simulink model "PTC_MBDS_DateTimeAssemble_Sample"  (R2013a)
settings: Solver=FixedStepDiscrete  StartTime=0.0  StopTime=Inf  FixedStep=0.01  RelTol=1e-3
libraries: PTC_MBDS_LIB x3, simulink_extras x2
settings Model: Creator=Jordan.Mosher  LastModifiedBy=Sundeep.Tuteja

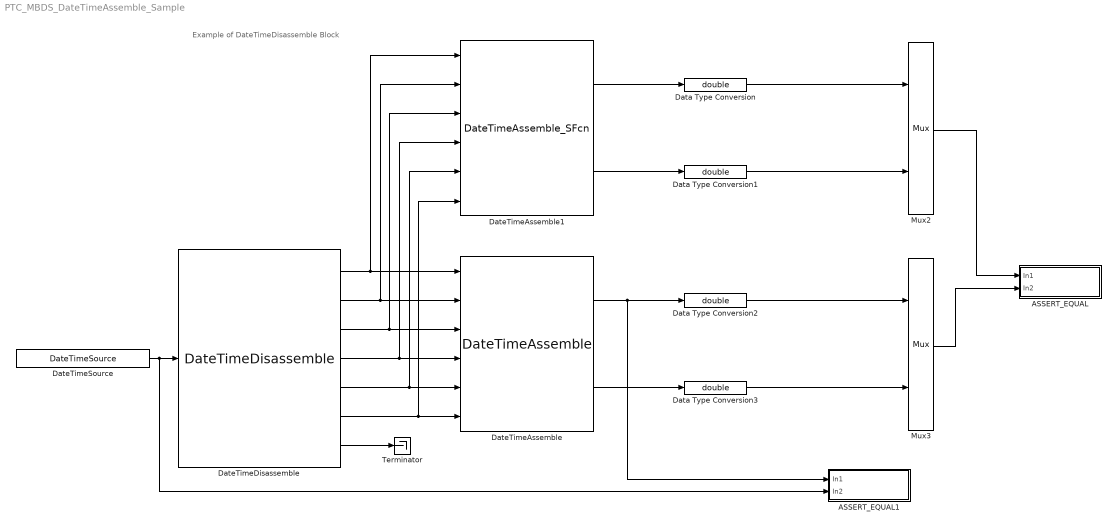
== system PTC_MBDS_DateTimeAssemble_Sample ==
  note: Example of DateTimeDisassemble Block
  ASSERT_EQUAL : Subsystem
  ASSERT_EQUAL1 : Subsystem
  Data Type Conversion{,1..3} (4 alike) : DataTypeConversion  OutDataTypeStr=double  SaturateOnIntegerOverflow=on
  DateTimeAssemble : PTC_MBDS_LIB/MBDS Standard Library/Extended Operations/Date & Time Operations/Date & Time Conversions/DateTimeAssemble  ENO_Enabled=on  PTC_MBDS_BlockVersion=5.40  PTC_BlockType=PTC_MBDS_DateTimeAssemble
  DateTimeAssemble1 : S-Function  InitFcn=|  FunctionName=DateTimeAssemble_SFcn  Parameters=boolean(ENO_Enabled)  EnableBusSupport=off  mask(DateTimeAssemble){MBDS_LibraryBlock=on, ENO_Enabled=on, MBDS_BlockVersion=05.40}
      | if(exist('MBDS_BlockCallback', 'file'))
      |    MBDS_BlockCallback('Update', gcb);  
      | end
      mask prompts: MBDS_LibraryBlock "MBDS Library Block"; ENO_Enabled "Show ENO port"; MBDS_BlockVersion "Block version:"
      mask help: Assembles a date_time signal from individual date and time components. The input values are restricted to their ranges (refer to the block help). If an input is out of range the ENO output is set to false.
      mask init:
      | MBDS_BlockCallback('Copy', gcb);     
      | maskdisplay = 'disp(sprintf(''Date Time\nAssemble''))';
      | maskdisplay = [maskdisplay 10 'port_label(''input'', 1, ''Year'')' 10];
      | maskdisplay = [maskdisplay 'port_label(''input'', 2, ''Month'')' 10];
      | maskdisplay = [maskdisplay 'port_label(''input'', 3, ''Day'')' 10];
      | maskdisplay = [maskdisplay 'port_label(''input'', 4, ''Hours'')' 10];
      | maskdisplay = [maskdisplay 'port_label(''input'', 5, ''Minutes'')' 10];
      | maskdisplay = [maskdisplay 'port_label(''input'', 6, ''Seconds'')' 10];
      | maskdisplay = [maskdisplay 'port_label(''output'', 1, ''DT'')' 10];
      | if(ENO_Enabled)
      |     maskdisplay = [maskdisplay 'port_label(''output'', 2, ''ENO'')' 10];
      | end
      | set_param(gcbh, 'maskdisplay', maskdisplay)
      mask Help: eval(['open([workdir(''RT_Dir:''),''\Host\Library\Blockset\Help\'',get_param(gcb,''MaskType''),''.html''])']);
      mask Display:
      | disp(sprintf('Date Time\nAssemble'))
      | port_label('input', 1, 'Year')
      | port_label('input', 2, 'Month')
      | port_label('input', 3, 'Day')
      | port_label('input', 4, 'Hours')
      | port_label('input', 5, 'Minutes')
      | port_label('input', 6, 'Seconds')
      | port_label('output', 1, 'DT')
      | port_label('output', 2, 'ENO')
  DateTimeDisassemble : PTC_MBDS_LIB/MBDS Standard Library/Extended Operations/Date & Time Operations/Date & Time Conversions/DateTimeDisassemble  ENO_Enabled=off  PTC_MBDS_BlockVersion=5.40  PTC_BlockType=PTC_MBDS_DateTimeDisassemble
  DateTimeSource : PTC_MBDS_LIB/MBDS Standard Library/Extended Operations/Date & Time Operations/DateTimeSource  InputValue=1986-12-01-12:55:13  PTC_MBDS_BlockVersion=5.40  PTC_BlockType=PTC_MBDS_DateTimeSource  Value=533825713
  Mux2 : Mux  Inputs=2
  Mux3 : Mux  Inputs=2
  Terminator : Terminator
      settings: InitFcn=|
      | try
      |    MBDS_BlockCallback('Update', gcb);
      | end
  wires:
  Mux3/1 -> ASSERT_EQUAL/2(In2)
  Mux2/1 -> ASSERT_EQUAL/1(In1)
  DateTimeDisassemble/7 -> Terminator/1
  DateTimeSource/1 -> ASSERT_EQUAL1/2(In2), DateTimeDisassemble/1
  DateTimeDisassemble/4 -> DateTimeAssemble1/4, DateTimeAssemble/4
  DateTimeDisassemble/5 -> DateTimeAssemble1/5, DateTimeAssemble/5
  DateTimeDisassemble/1 -> DateTimeAssemble1/1, DateTimeAssemble/1
  DateTimeDisassemble/2 -> DateTimeAssemble1/2, DateTimeAssemble/2
  DateTimeDisassemble/3 -> DateTimeAssemble1/3, DateTimeAssemble/3
  DateTimeDisassemble/6 -> DateTimeAssemble1/6, DateTimeAssemble/6
  DateTimeAssemble1/1 -> Data Type Conversion/1
  DateTimeAssemble1/2 -> Data Type Conversion1/1
  DateTimeAssemble/2 -> Data Type Conversion3/1
  DateTimeAssemble/1 -> ASSERT_EQUAL1/1(In1), Data Type Conversion2/1
  Data Type Conversion/1 -> Mux2/1
  Data Type Conversion1/1 -> Mux2/2
  Data Type Conversion2/1 -> Mux3/1
  Data Type Conversion3/1 -> Mux3/2

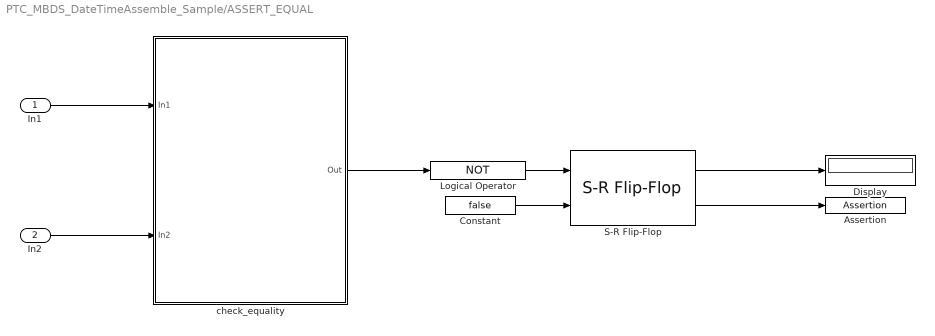
== system PTC_MBDS_DateTimeAssemble_Sample/ASSERT_EQUAL ==
  In1 : Inport
  In2 : Inport  Port=2
  Assertion : Assertion
  Constant : Constant  Value=false
  Display : Display
  Logical Operator : Logic  Operator=NOT  AllPortsSameDT=off  OutDataTypeStr=boolean
  S-R Flip-Flop : simulink_extras/Flip Flops/S-R Flip-Flop  initial_condition=0
  check_equality : MATLAB Function  TreatAsAtomicUnit=on
  wires:
  S-R Flip-Flop/1 -> Display/1
  check_equality/1(Out) -> Logical Operator/1
  Constant/1 -> S-R Flip-Flop/2
  S-R Flip-Flop/2 -> Assertion/1
  In2/1 -> check_equality/2(In2)
  In1/1 -> check_equality/1(In1)
  Logical Operator/1 -> S-R Flip-Flop/1

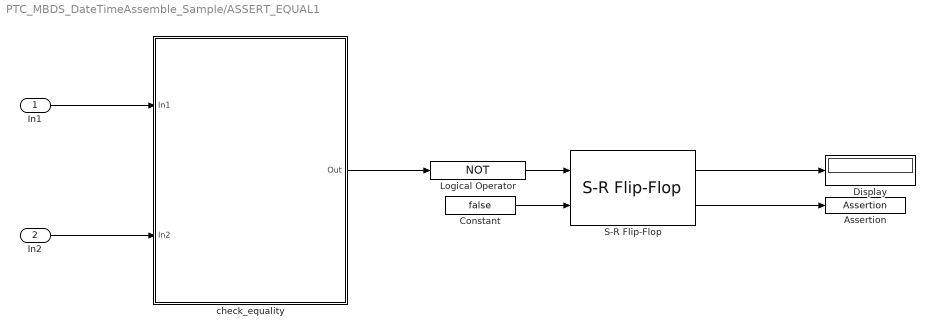
== system PTC_MBDS_DateTimeAssemble_Sample/ASSERT_EQUAL1 ==
  In1 : Inport
  In2 : Inport  Port=2
  Assertion : Assertion
  Constant : Constant  Value=false
  Display : Display
  Logical Operator : Logic  Operator=NOT  AllPortsSameDT=off  OutDataTypeStr=boolean
  S-R Flip-Flop : simulink_extras/Flip Flops/S-R Flip-Flop  initial_condition=0
  check_equality : MATLAB Function  TreatAsAtomicUnit=on
  wires:
  Logical Operator/1 -> S-R Flip-Flop/1
  In1/1 -> check_equality/1(In1)
  In2/1 -> check_equality/2(In2)
  S-R Flip-Flop/2 -> Assertion/1
  Constant/1 -> S-R Flip-Flop/2
  check_equality/1(Out) -> Logical Operator/1
  S-R Flip-Flop/1 -> Display/1

== matlab function PTC_MBDS_DateTimeAssemble_Sample/ASSERT_EQUAL1/check_equality ==
  data: In1 input; Out output; In2 input
function Out = check_equality(In1, In2)
%#codegen

Out = isequaln(In1, In2);

end

== matlab function PTC_MBDS_DateTimeAssemble_Sample/ASSERT_EQUAL/check_equality ==
  data: In1 input; Out output; In2 input
function Out = check_equality(In1, In2)
%#codegen

Out = isequaln(In1, In2);

end
